simulink model "AustMechanicalModel"  (R2018a)
settings: Solver=FixedStepAuto  StartTime=0.0  StopTime=10.0  FixedStep=10e-4  RelTol=1e-3
values from neighbouring files (symbols this model uses):
  martFrac = martStressFrac + martTempFrac    (= 1)    [AustRunner.m]
  martStressFrac = 1    [AustRunner.m]
  martTempFrac = 0    [AustRunner.m]
  strainZero = rEmax    [AustRunner.m]
  stressParam = stress_range(i)    [AustRunner.m]
  tempFinish = 100    [AustRunner.m]
  tempStart = As - 273    [AustRunner.m]
undefined symbols (not defined in the file or in its folder): Af, As, Ca, Da, Dm, rEmax, Theta
settings Model: Creator=Michau  LastModifiedBy=Michau

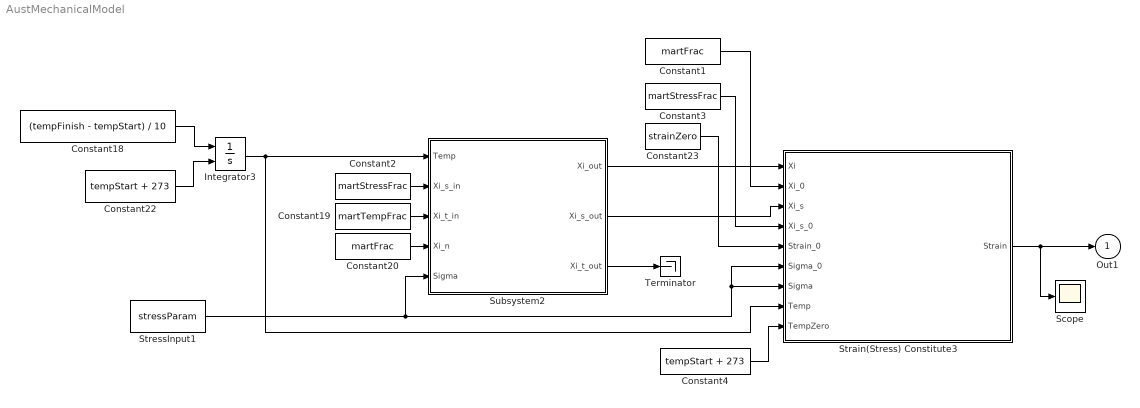
== system AustMechanicalModel ==
  Constant1 : Constant  Value=martFrac
  Constant18 : Constant  Value=(tempFinish - tempStart) / 10
  Constant19 : Constant  Value=martTempFrac
  Constant2 : Constant  Value=martStressFrac
  Constant20 : Constant  Value=martFrac
  Constant22 : Constant  Value=tempStart + 273
  Constant23 : Constant  Value=strainZero
  Constant3 : Constant  Value=martStressFrac
  Constant4 : Constant  Value=tempStart + 273
  Integrator3 : Integrator  InitialConditionSource=external
  Scope : Scope
  Strain(Stress) Constitute3 : Subsystem
  StressInput1 : Constant  Value=stressParam
  Subsystem2 : Subsystem
  Terminator : Terminator
  Out1 : Outport
  wires:
  Subsystem2/1(Xi_out) -> Strain(Stress) Constitute3/1(Xi)
  Constant2/1 -> Subsystem2/2(Xi_s_in)
  Constant1/1 -> Strain(Stress) Constitute3/2(Xi_0)
  Constant19/1 -> Subsystem2/3(Xi_t_in)
  Constant20/1 -> Subsystem2/4(Xi_n)
  Constant23/1 -> Strain(Stress) Constitute3/5(Strain_0)
  Constant22/1 -> Integrator3/2
  Integrator3/1 -> Strain(Stress) Constitute3/8(Temp), Subsystem2/1(Temp)
  Strain(Stress) Constitute3/1(Strain) -> Scope/1, Out1/1
  Subsystem2/2(Xi_s_out) -> Strain(Stress) Constitute3/3(Xi_s)
  Constant3/1 -> Strain(Stress) Constitute3/4(Xi_s_0)
  Constant18/1 -> Integrator3/1
  StressInput1/1 -> Subsystem2/5(Sigma), Strain(Stress) Constitute3/6(Sigma_0), Strain(Stress) Constitute3/7(Sigma)
  Subsystem2/3(Xi_t_out) -> Terminator/1
  Constant4/1 -> Strain(Stress) Constitute3/9(TempZero)

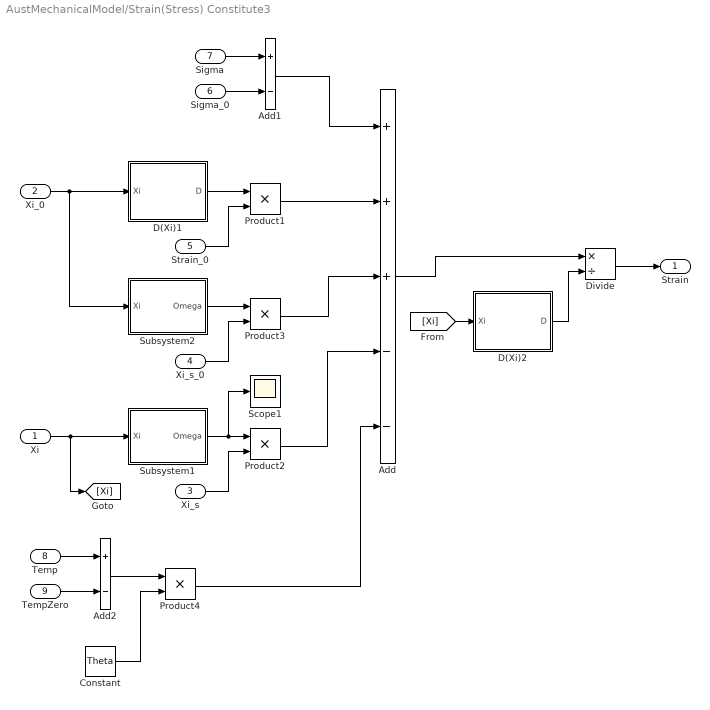
== system AustMechanicalModel/Strain(Stress) Constitute3 ==
  Xi : Inport
  Xi_0 : Inport  Port=2
  Xi_s : Inport  Port=3
  Xi_s_0 : Inport  Port=4
  Strain_0 : Inport  Port=5
  Sigma_0 : Inport  Port=6
  Sigma : Inport  Port=7
  Temp : Inport  Port=8
  TempZero : Inport  Port=9
  Add : Sum  Inputs=+++--
  Add1 : Sum  Inputs=+-
  Add2 : Sum  Inputs=+-
  Constant : Constant  Value=Theta
  D(Xi)1 : Subsystem
  D(Xi)2 : Subsystem
  Divide : Product  Inputs=*/
  Product{1..4} (4 alike) : Product
  Scope1 : Scope
  Subsystem1 : Subsystem
  Subsystem2 : Subsystem
  Strain : Outport
  wires:
  D(Xi)1/1(D) -> Product1/1
  Strain_0/1 -> Product1/2
  Xi/1 -> Subsystem1/1(Xi), [Xi]
  Subsystem1/1(Omega) -> Scope1/1, Product2/1
  Xi_0/1 -> Subsystem2/1(Xi), D(Xi)1/1(Xi)
  Subsystem2/1(Omega) -> Product3/1
  Xi_s_0/1 -> Product3/2
  Add/1 -> Divide/1
  Sigma_0/1 -> Add1/2
  Sigma/1 -> Add1/1
  Add1/1 -> Add/1
  Xi_s/1 -> Product2/2
  Product1/1 -> Add/2
  Product3/1 -> Add/3
  Product2/1 -> Add/4
  [Xi] -> D(Xi)2/1(Xi)
  D(Xi)2/1(D) -> Divide/2
  Divide/1 -> Strain/1
  Temp/1 -> Add2/1
  TempZero/1 -> Add2/2
  Add2/1 -> Product4/1
  Constant/1 -> Product4/2
  Product4/1 -> Add/5

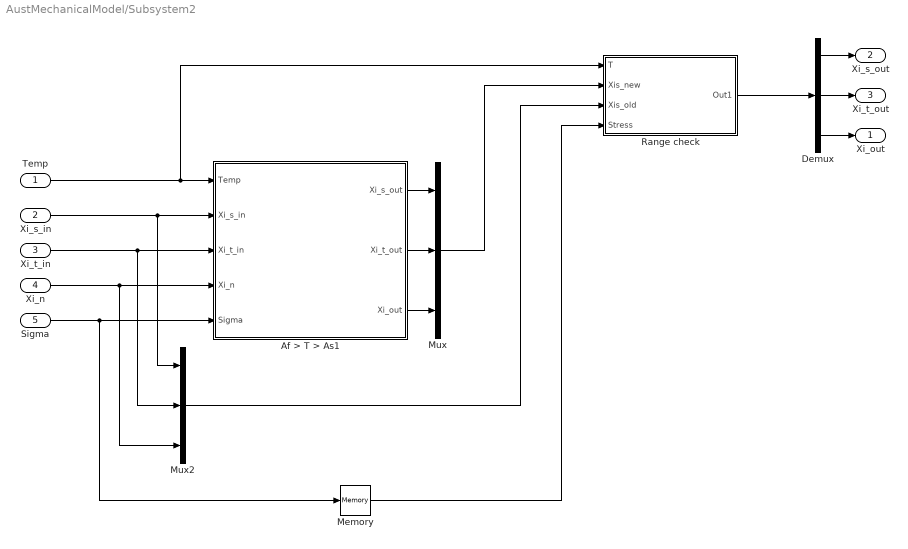
== system AustMechanicalModel/Subsystem2 ==
  Temp : Inport
  Xi_s_in : Inport  Port=2
  Xi_t_in : Inport  Port=3
  Xi_n : Inport  Port=4
  Sigma : Inport  Port=5
  Af > T > As1 : Subsystem
  Demux : Demux  Outputs=3
  Memory : Memory
  Mux : Mux  Inputs=3
  Mux2 : Mux  Inputs=3
  Range check : Subsystem
  Xi_out : Outport
  Xi_s_out : Outport  Port=2
  Xi_t_out : Outport  Port=3
  wires:
  Af > T > As1/2(Xi_t_out) -> Mux/2
  Af > T > As1/3(Xi_out) -> Mux/3
  Sigma/1 -> Memory/1, Af > T > As1/5(Sigma)
  Temp/1 -> Range check/1(T), Af > T > As1/1(Temp)
  Xi_n/1 -> Mux2/3, Af > T > As1/4(Xi_n)
  Xi_s_in/1 -> Mux2/1, Af > T > As1/2(Xi_s_in)
  Xi_t_in/1 -> Mux2/2, Af > T > As1/3(Xi_t_in)
  Af > T > As1/1(Xi_s_out) -> Mux/1
  Demux/1 -> Xi_s_out/1
  Demux/2 -> Xi_t_out/1
  Demux/3 -> Xi_out/1
  Mux/1 -> Range check/2(Xis_new)
  Mux2/1 -> Range check/3(Xis_old)
  Range check/1(Out1) -> Demux/1
  Memory/1 -> Range check/4(Stress)

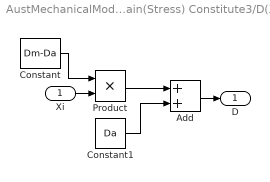
== system AustMechanicalModel/Strain(Stress) Constitute3/D(Xi)1 ==
  Xi : Inport
  Add : Sum
  Constant : Constant  Value=Dm-Da
  Constant1 : Constant  Value=Da
  Product : Product
  D : Outport
  wires:
  Xi/1 -> Product/2
  Product/1 -> Add/1
  Constant1/1 -> Add/2
  Constant/1 -> Product/1
  Add/1 -> D/1

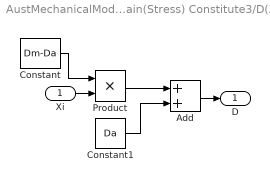
== system AustMechanicalModel/Strain(Stress) Constitute3/D(Xi)2 ==
  Xi : Inport
  Add : Sum
  Constant : Constant  Value=Dm-Da
  Constant1 : Constant  Value=Da
  Product : Product
  D : Outport
  wires:
  Xi/1 -> Product/2
  Product/1 -> Add/1
  Constant1/1 -> Add/2
  Constant/1 -> Product/1
  Add/1 -> D/1

== system AustMechanicalModel/Strain(Stress) Constitute3/Subsystem1 ==
  Xi : Inport
  Constant : Constant  Value=-rEmax
  Product : Product
  Subsystem1 : Subsystem
  Omega : Outport
  wires:
  Product/1 -> Omega/1
  Subsystem1/1(D) -> Product/1
  Constant/1 -> Product/2
  Xi/1 -> Subsystem1/1(Xi)

== system AustMechanicalModel/Strain(Stress) Constitute3/Subsystem2 ==
  Xi : Inport
  Constant : Constant  Value=-rEmax
  Product : Product
  Subsystem1 : Subsystem
  Omega : Outport
  wires:
  Product/1 -> Omega/1
  Subsystem1/1(D) -> Product/1
  Constant/1 -> Product/2
  Xi/1 -> Subsystem1/1(Xi)

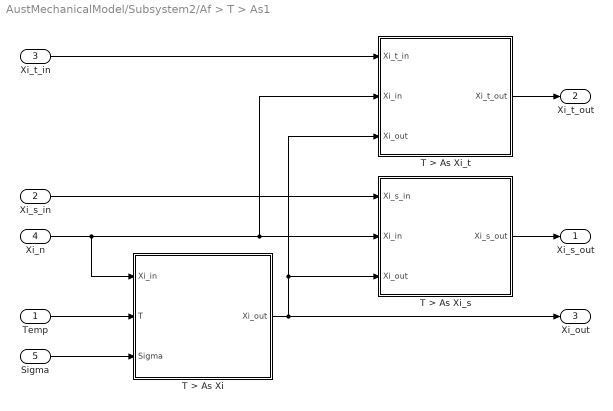
== system AustMechanicalModel/Subsystem2/Af > T > As1 ==
  Temp : Inport
  Xi_s_in : Inport  Port=2
  Xi_t_in : Inport  Port=3
  Xi_n : Inport  Port=4
  Sigma : Inport  Port=5
  "T > As Xi " : Subsystem
  T > As Xi_s : Subsystem
  T > As Xi_t : Subsystem
  Xi_s_out : Outport
  Xi_t_out : Outport  Port=2
  Xi_out : Outport  Port=3
  wires:
  Sigma/1 -> "T > As Xi "/3("Sigma ")
  "T > As Xi "/1(Xi_out) -> T > As Xi_s/3(Xi_out), T > As Xi_t/3(Xi_out), Xi_out/1
  Xi_s_in/1 -> T > As Xi_s/1("Xi_s_in ")
  Xi_n/1 -> "T > As Xi "/1(Xi_in), T > As Xi_t/2(Xi_in), T > As Xi_s/2(Xi_in)
  T > As Xi_s/1(Xi_s_out) -> Xi_s_out/1
  Temp/1 -> "T > As Xi "/2(T)
  Xi_t_in/1 -> T > As Xi_t/1("Xi_t_in ")
  T > As Xi_t/1(Xi_t_out) -> Xi_t_out/1

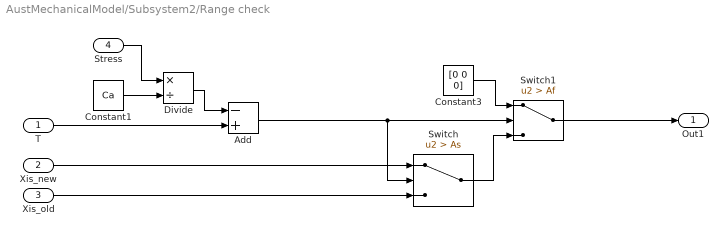
== system AustMechanicalModel/Subsystem2/Range check ==
  T : Inport
  Xis_new : Inport  Port=2
  Xis_old : Inport  Port=3
  Stress : Inport  Port=4
  Add : Sum  Inputs=-+
  Constant1 : Constant  Value=Ca
  Constant3 : Constant  Value=[0 0 0]
  Divide : Product  Inputs=*/
  Switch : Switch  Criteria=u2 > Threshold  Threshold=As
  Switch1 : Switch  Criteria=u2 > Threshold  Threshold=Af
  Out1 : Outport
  wires:
  Switch/1 -> Switch1/3
  Constant3/1 -> Switch1/1
  Xis_old/1 -> Switch/3
  T/1 -> Add/2
  Xis_new/1 -> Switch/1
  Switch1/1 -> Out1/1
  Add/1 -> Switch/2, Switch1/2
  Stress/1 -> Divide/1
  Constant1/1 -> Divide/2
  Divide/1 -> Add/1

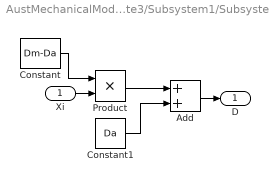
== system AustMechanicalModel/Strain(Stress) Constitute3/Subsystem1/Subsystem1 ==
  Xi : Inport
  Add : Sum
  Constant : Constant  Value=Dm-Da
  Constant1 : Constant  Value=Da
  Product : Product
  D : Outport
  wires:
  Xi/1 -> Product/2
  Product/1 -> Add/1
  Constant1/1 -> Add/2
  Constant/1 -> Product/1
  Add/1 -> D/1

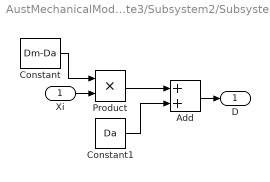
== system AustMechanicalModel/Strain(Stress) Constitute3/Subsystem2/Subsystem1 ==
  Xi : Inport
  Add : Sum
  Constant : Constant  Value=Dm-Da
  Constant1 : Constant  Value=Da
  Product : Product
  D : Outport
  wires:
  Xi/1 -> Product/2
  Product/1 -> Add/1
  Constant1/1 -> Add/2
  Constant/1 -> Product/1
  Add/1 -> D/1

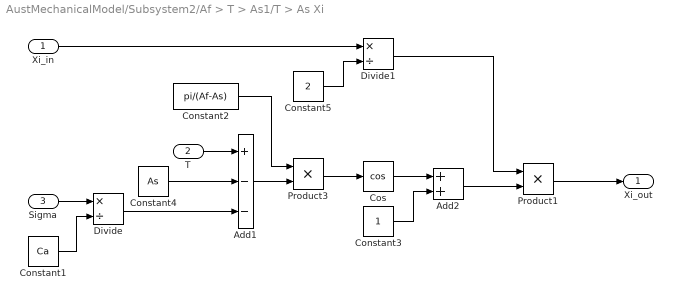
== system AustMechanicalModel/Subsystem2/Af > T > As1/T > As Xi  ==
  Xi_in : Inport
  T : Inport  Port=2
  "Sigma " : Inport  Port=3
  Add1 : Sum  Inputs=+--
  Add2 : Sum
  Constant1 : Constant  Value=Ca
  Constant2 : Constant  Value=pi/(Af-As)
  Constant3 : Constant
  Constant4 : Constant  Value=As
  Constant5 : Constant  Value=2
  Cos : Trigonometry  Operator=cos
  Divide : Product  Inputs=*/
  Divide1 : Product  Inputs=*/
  Product1 : Product
  Product3 : Product
  Xi_out : Outport
  wires:
  Constant4/1 -> Add1/2
  Xi_in/1 -> Divide1/1
  T/1 -> Add1/1
  Add1/1 -> Product3/2
  Constant2/1 -> Product3/1
  Product3/1 -> Cos/1
  "Sigma "/1 -> Divide/1
  Constant1/1 -> Divide/2
  Divide/1 -> Add1/3
  Cos/1 -> Add2/1
  Constant3/1 -> Add2/2
  Constant5/1 -> Divide1/2
  Add2/1 -> Product1/2
  Divide1/1 -> Product1/1
  Product1/1 -> Xi_out/1

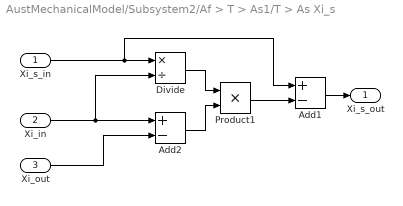
== system AustMechanicalModel/Subsystem2/Af > T > As1/T > As Xi_s ==
  "Xi_s_in " : Inport
  Xi_in : Inport  Port=2
  Xi_out : Inport  Port=3
  Add1 : Sum  Inputs=+-
  Add2 : Sum  Inputs=+-
  Divide : Product  Inputs=*/
  Product1 : Product
  Xi_s_out : Outport
  wires:
  Xi_in/1 -> Add2/1, Divide/2
  "Xi_s_in "/1 -> Add1/1, Divide/1
  Add1/1 -> Xi_s_out/1
  Xi_out/1 -> Add2/2
  Divide/1 -> Product1/1
  Add2/1 -> Product1/2
  Product1/1 -> Add1/2

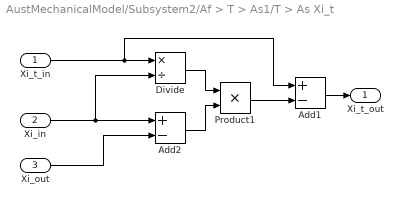
== system AustMechanicalModel/Subsystem2/Af > T > As1/T > As Xi_t ==
  "Xi_t_in " : Inport
  Xi_in : Inport  Port=2
  Xi_out : Inport  Port=3
  Add1 : Sum  Inputs=+-
  Add2 : Sum  Inputs=+-
  Divide : Product  Inputs=*/
  Product1 : Product
  Xi_t_out : Outport
  wires:
  Xi_in/1 -> Add2/1, Divide/2
  "Xi_t_in "/1 -> Add1/1, Divide/1
  Add1/1 -> Xi_t_out/1
  Xi_out/1 -> Add2/2
  Divide/1 -> Product1/1
  Add2/1 -> Product1/2
  Product1/1 -> Add1/2
